simulink model "A_ZH_Z5"  (R2025a)
settings: Solver=ode45  StartTime=0.0  StopTime=10  RelTol=1e-3  EnableMultiTasking=on
settings Model: Creator=oktato  LastModifiedBy=Szalay
settings SolverCC: AlgebraicLoopSolver=TrustRegion
settings DataIOCC: LimitDataPoints=on  SaveFormat=Array  ReturnWorkspaceOutputs=off
settings OptimizationCC: LifeSpan=inf
settings DebuggingCC: UnderspecifiedInitializationDetection=Classic  MergeDetectMultiDrivingBlocksExec=none  SolverPrmCheckMsg=warning  UnconnectedInputMsg=warning  UnconnectedOutputMsg=warning  UnconnectedLineMsg=warning  SFUnexpectedBacktrackingDiag=warning  SFNoUnconditionalDefaultTransitionDiag=warning  SFExecutionAtInitializationDiag=none  ArithmeticOperatorsInVariantConditions=warning
settings HardwareCC: ProdBitPerPointer=32.0  ProdBitPerSizeT=32.0  ProdBitPerPtrDiffT=32.0  ProdLargestAtomicFloat=None  ProdIntDivRoundTo=Undefined  ProdEndianess=Unspecified  ProdWordSize=32.0  ProdHWDeviceType=32-bit Generic
settings ModelReferenceCC: PropagateSignalLabelsOutOfModel=off
settings SFSimCC: SimUseLocalCustomCode=off  CustomCodeUndefinedFunction=UseInterfaceOnly
settings RTWCC: RTWUseLocalCustomCode=off  GPUComputeCapability=3.5
settings CodeAppCC: StateflowObjectComments=on
settings GRTTargetCC: TargetLangStandard=C89/C90 (ANSI)
settings ConfigComp: CovMetricSettings=dw  CovSaveCumulativeToWorkspaceVar=on  CovSaveSingleToWorkspaceVar=on  CovExternalEMLEnable=off

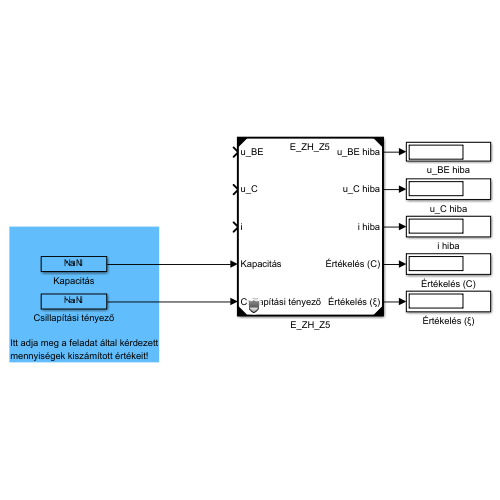
[thumbnail: Simulink's stored preview of the top-level diagram]
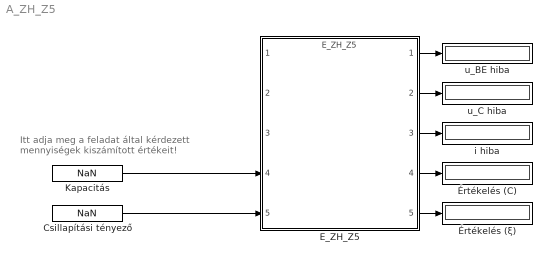
== system A_ZH_Z5 ==
  note: Itt adja meg a feladat által kérdezett
      | mennyiségek kiszámított értékeit!
  Csillapítási tényező : Constant  Value=NaN
  E_ZH_Z5 : ModelReference  ModelNameDialog=E_ZH_Z5.slxp  ModelReferenceVersion=1.13  CopyOfModelProtected=on
  Kapacitás : Constant  Value=NaN
  i hiba : Display
  u_BE hiba : Display
  u_C hiba : Display
  Értékelés (C) : Display
  Értékelés (ξ) : Display
  wires:
  E_ZH_Z5/3 -> i hiba/1
  E_ZH_Z5/1 -> u_BE hiba/1
  E_ZH_Z5/2 -> u_C hiba/1
  Kapacitás/1 -> E_ZH_Z5/4
  Csillapítási tényező/1 -> E_ZH_Z5/5
  E_ZH_Z5/5 -> Értékelés (ξ)/1
  E_ZH_Z5/4 -> Értékelés (C)/1
